simulink library "INT_Prp_TrqLeadCoord"  (R2016b)
settings: Solver=VariableStepAuto  StartTime=0.0  StopTime=10.0  RelTol=1e-3
settings Model: Creator=Administrator  LastModifiedBy=Administrator

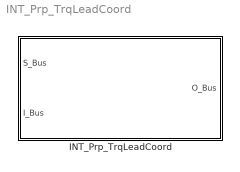
== system INT_Prp_TrqLeadCoord ==
  INT_Prp_TrqLeadCoord : Subsystem

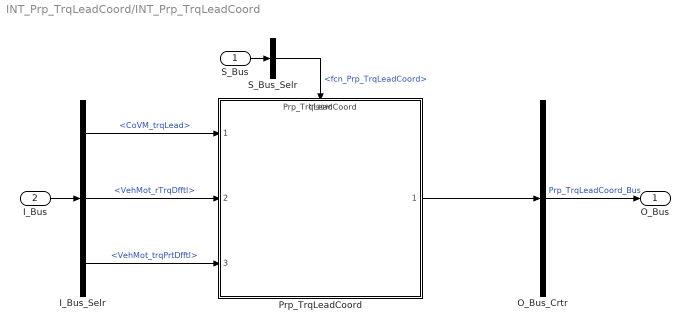
== system INT_Prp_TrqLeadCoord/INT_Prp_TrqLeadCoord ==
  S_Bus : Inport
  I_Bus : Inport  Port=2
  I_Bus_Selr : BusSelector  OutputSignals=CoVM_trqLead,VehMot_rTrqDfftl,VehMot_trqPrtDfftl
  O_Bus_Crtr : BusCreator  Inputs=1
  Prp_TrqLeadCoord : ModelReference  ModelNameDialog=Prp_TrqLeadCoord  SimulationMode=Normal  ModelReferenceVersion=1.6  TriggerPortName=function  TriggerPortTriggerType=function-call  TriggerPortStatesWhenEnabling=held
  S_Bus_Selr : BusSelector  OutputSignals=fcn_Prp_TrqLeadCoord
  O_Bus : Outport
  wires:
  S_Bus_Selr/1 -> Prp_TrqLeadCoord/Trigger  "<fcn_Prp_TrqLeadCoord>"
  S_Bus/1 -> S_Bus_Selr/1
  I_Bus/1 -> I_Bus_Selr/1
  I_Bus_Selr/1 -> Prp_TrqLeadCoord/1  "<CoVM_trqLead>"
  I_Bus_Selr/2 -> Prp_TrqLeadCoord/2  "<VehMot_rTrqDfftl>"
  I_Bus_Selr/3 -> Prp_TrqLeadCoord/3  "<VehMot_trqPrtDfftl>"
  O_Bus_Crtr/1 -> O_Bus/1  "Prp_TrqLeadCoord_Bus"
  Prp_TrqLeadCoord/1 -> O_Bus_Crtr/1
